simulink library "headingSetpointLookup_ul"  (R2018a)
settings: Solver=VariableStepAuto  StartTime=0.0  StopTime=10.0  RelTol=1e-3
values from neighbouring files (symbols this model uses):
  headingSetpointLookup = []    [headingSetpointLookup_ul_init.m]
  pathPositionLookup = []    [headingSetpointLookup_ul_init.m]
libraries: simulink x1
settings Model: Creator=mcobb  LastModifiedBy=mcobb

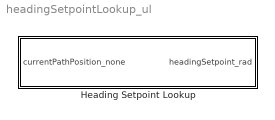
== system headingSetpointLookup_ul ==
  Heading Setpoint Lookup : Subsystem

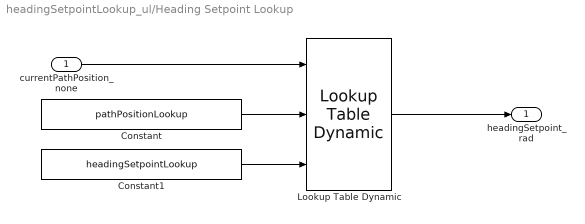
== system headingSetpointLookup_ul/Heading Setpoint Lookup ==
  currentPathPosition_none : Inport
  Constant : Constant  Value=pathPositionLookup
  Constant1 : Constant  Value=headingSetpointLookup
  Lookup Table Dynamic : simulink/Lookup Tables/Lookup Table Dynamic  LookUpMeth=Interpolation-Use End Values  OutDataType=fixdt('double')  OutScaling=2^-10  OutputDataTypeScalingMode=Specify via dialog  OutDataTypeStr=double  DoSatur=off
      settings: SourceProductName=Simulink
  headingSetpoint_rad : Outport
  wires:
  currentPathPosition_none/1 -> Lookup Table Dynamic/1
  Lookup Table Dynamic/1 -> headingSetpoint_rad/1
  Constant/1 -> Lookup Table Dynamic/2
  Constant1/1 -> Lookup Table Dynamic/3
